simulink model "Task_15"  (R2019b)
settings: Solver=ode23s  StartTime=0.0  StopTime=0.001  MaxStep=50e-9  RelTol=10e-6
undefined symbols (not defined in the file or in its folder): plecs
settings Model: Creator=Mariam  LastModifiedBy=Nahid
settings DataIOCC: ReturnWorkspaceOutputs=off
settings DebuggingCC: ArithmeticOperatorsInVariantConditions=warning
settings SFSimCC: CustomCodeUndefinedFunction=UseInterfaceOnly

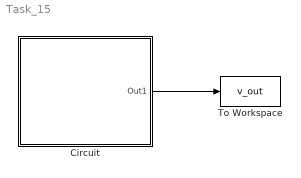
== system Task_15 ==
  Circuit : Subsystem  LoadFcn=plecs('sl', 200);  InitFcn=plecs('sl', 214);  StartFcn=plecs('sl', 208);  StopFcn=plecs('sl', 209);  mask(PlecsCircuit){PLECSData=<binary blob, 5424 chars, not shown>}
      mask prompts: PLECSData "PLECS Data (Do not delete or modify!)"
      mask init:
      | % PLACE CUSTOM INITIALIZATIONS ABOVE
      | % DO NOT REMOVE
      | plecs('sl', 215);
      | % DO NOT REMOVE
      settings: CopyFcn=plecs('sl', 203);  DeleteFcn=plecs('sl', 205);  UndoDeleteFcn=plecs('sl', 206);  PreSaveFcn=plecs('sl', 211);  PostSaveFcn=plecs('sl', 201);  NameChangeFcn=plecs('sl', 210);  DestroyFcn=plecs('sl', 207);  PreCopyFcn=plecs('sl', 216);  OpenFcn=plecs('sl', 202);  ErrorFcn=plerrorfcn
      mask Help: web(['file:///' fullfile(plecsdoc, 'creatingacircuit.html')])
      mask Display: disp('PLECS\nCircuit')
  To Workspace : ToWorkspace  VariableName=v_out  SampleTime=-1
      settings: MaxDataPoints=1
  wires:
  Circuit/1(Out1) -> To Workspace/1

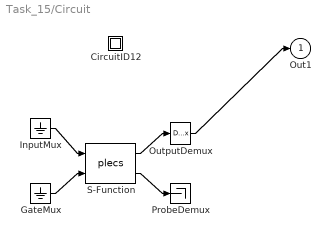
== system Task_15/Circuit ==
  " CircuitID12 " : Subsystem
  " GateMux " : Ground
  " InputMux " : Ground
  " OutputDemux " : Demux  Outputs=[ 1 ]
  " ProbeDemux " : Terminator
  " S-Function " : S-Function  FunctionName=plecs  SFunctionDeploymentMode=off  EnableBusSupport=off
  Out1 : Outport  PortDimensions=1  VectorParamsAs1DForOutWhenUnconnected=off
  wires:
  " InputMux "/1 -> " S-Function "/1
  " GateMux "/1 -> " S-Function "/2
  " S-Function "/1 -> " OutputDemux "/1
  " S-Function "/2 -> " ProbeDemux "/1
  " OutputDemux "/1 -> Out1/1

== system Task_15/Circuit/ CircuitID12  ==
